simulink model "flattening"  (Simulink 7.9)
settings: Solver=ode45  StartTime=0.0  StopTime=10.0  RelTol=1e-3
undefined symbols (not defined in the file or in its folder): ARULE, TransformationLib
libraries: Pre_CommonlyUsedBlocks x5, Post_CommonlyUsedBlocks x3
settings Model: Creator=jdenil  LastModifiedBy=boakes

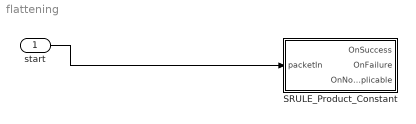
== system flattening ==
  start : Inport
  SRULE_Product_Constant : Subsystem  AncestorBlock=TransformationLib/ARULE
  wires:
  start/1 -> SRULE_Product_Constant/1(packetIn)

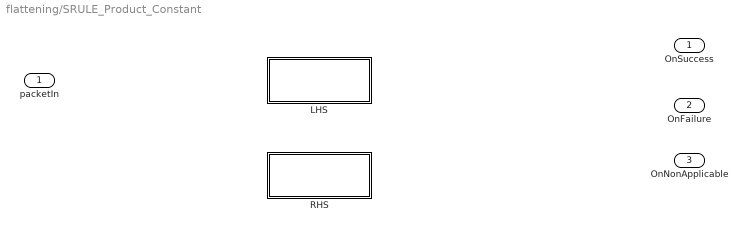
== system flattening/SRULE_Product_Constant ==
  packetIn : Inport
  LHS : Subsystem
  RHS : Subsystem
  OnSuccess : Outport
  OnFailure : Outport  Port=2
  OnNonApplicable : Outport  Port=3

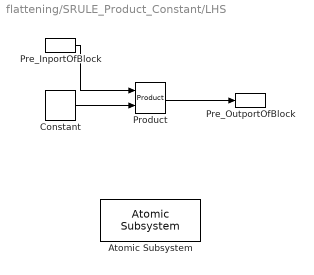
== system flattening/SRULE_Product_Constant/LHS ==
  Atomic Subsystem : Pre_CommonlyUsedBlocks/Atomic Subsystem  p_label=10  pre_Name=return True  pre_Position=return True
      settings: AttributesFormatString=%<p_label>
  Constant : Pre_CommonlyUsedBlocks/Constant  pre_label=1  pre_value=return True  pre_Name=return True  pre_Position=return True
      settings: AttributesFormatString=%<pre_label>
  Pre_InportOfBlock : Pre_CommonlyUsedBlocks/Pre_InportOfBlock  pre_label=0
      settings: AttributesFormatString=%<pre_label>
  Pre_OutportOfBlock : Pre_CommonlyUsedBlocks/Pre_OutportOfBlock  pre_label=4
      settings: AttributesFormatString=%<pre_label>
  Product : Pre_CommonlyUsedBlocks/Product  pre_label=2  pre_Name=return True  pre_Position=return True
      settings: AttributesFormatString=%<pre_label>
  wires:
  Pre_InportOfBlock/1 -> Product/1
  Constant/1 -> Product/2
  Product/1 -> Pre_OutportOfBlock/1

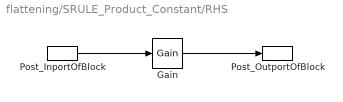
== system flattening/SRULE_Product_Constant/RHS ==
  Gain : Post_CommonlyUsedBlocks/Gain  post_label=5  post_gain=return PreNode('1')['value']  post_Name=return PreNode('1')['Name']+'Gain'  post_Position=return PreNode('1')['Position']
      settings: AttributesFormatString=%<post_label>
  Post_InportOfBlock : Post_CommonlyUsedBlocks/Post_InportOfBlock  post_label=0
      settings: AttributesFormatString=%<post_label>
  Post_OutportOfBlock : Post_CommonlyUsedBlocks/Post_OutportOfBlock  post_label=4
      settings: AttributesFormatString=%<post_label>
  wires:
  Post_InportOfBlock/1 -> Gain/1
  Gain/1 -> Post_OutportOfBlock/1
